simulink model "quad_reaction_wheel_controller"  (R2025b)
settings: Solver=VariableStepAuto  StartTime=0.0  StopTime=10.0  RelTol=1e-3
undefined symbols (not defined in the file): Kd, Kp
settings Model: Creator=taizo  LastModifiedBy=taizo

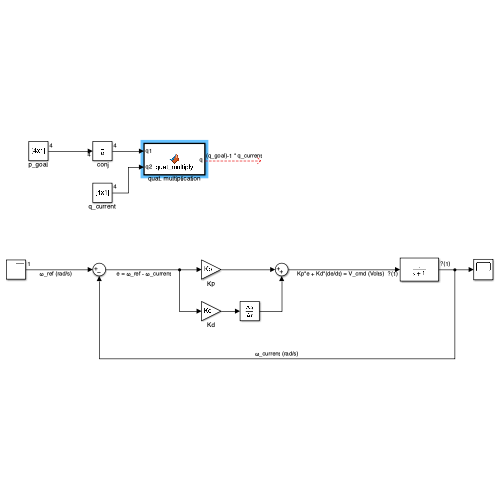
[thumbnail: Simulink's stored preview of the top-level diagram]
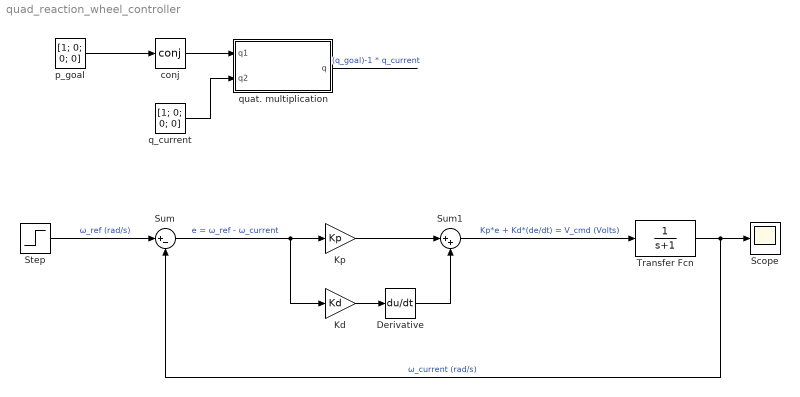
== system quad_reaction_wheel_controller ==
  " conj" : Math  Operator=conj
  Derivative : Derivative
  Kd : Gain  Gain=Kd
  Kp : Gain  Gain=Kp
  Scope : Scope
      settings: ActiveDisplayYMinimum=-0.06249  ActiveDisplayYMaximum=0.56242
  Step : Step  SampleTime=0
  Sum : Sum  Inputs=|+-
  Sum1 : Sum  Inputs=|++
  Transfer Fcn : TransferFcn  Denominator=[1 1]
  p_goal : Constant  Value=[1; 0; 0; 0]
  q_current : Constant  Value=[1; 0; 0; 0]
  quat. multiplication : MATLAB Function  TreatAsAtomicUnit=on
  wires:
  Step/1 -> Sum/1  "ω_ref (rad/s)"
  Derivative/1 -> Sum1/2
  Kp/1 -> Sum1/1
  Sum/1 -> Kd/1, Kp/1  "e = ω_ref - ω_current"
  Sum1/1 -> Transfer Fcn/1  "Kp*e + Kd*(de/dt) = V_cmd (Volts)"
  Transfer Fcn/1 -> Sum/2, Scope/1  "ω_current (rad/s)"
  Kd/1 -> Derivative/1
  p_goal/1 -> " conj"/1
  q_current/1 -> quat. multiplication/2(q2)
  quat. multiplication/1(q) -> ?  "(q_goal)-1 * q_current"
  " conj"/1 -> quat. multiplication/1(q1)

== matlab function quad_reaction_wheel_controller/quat. multiplication ==
  data: q1 input; q output; q2 input
function q = quat_multiply(q1, q2)

q0 = q1(1)*q2(1) - dot(q1(2:4), q2(2:4));

%explicitly
q1 = q2(1)*q1(2) + q2(2)*q1(1) - q2(3)*q1(4) + q2(4)*q1(3);
q2 = q2(1)*q1(3) + q2(2)*q1(4) + q2(3)*q1(1) - q2(4)*q1(2);
q3 = q2(1)*q1(4) - q2(2)*q1(3) + q2(3)*q1(2) + q2(4)*q1(1);

q = [q0; q1; q2; q3];

%chat

% qv = q1(1)*q2(2:4)...
%    + q2(1)*q1(2:4)...
%    + cross(q1(2:4), q2(2:4));
% 
% q = [q0; qv(:)];
